simulink model "Fierro_seguidor"  (R2018a)
settings: Solver=ode45  StartTime=0.0  StopTime=1  RelTol=1e-5  EnableMultiTasking=on
undefined symbols (not defined in the file): KIm, Km, KPm, Pm
libraries: simulink x3
settings Model: Creator=dwbertol  LastModifiedBy=bruno
settings DataIOCC: LimitDataPoints=on  SaveFormat=Array  SignalLoggingSaveFormat=ModelDataLogs
settings OptimizationCC: ExpressionDepthLimit=2147483647  LifeSpan=inf
settings DebuggingCC: UnderspecifiedInitializationDetection=Classic  MergeDetectMultiDrivingBlocksExec=none  SolverPrmCheckMsg=warning  FcnCallInpInsideContextMsg=warning  StateNameClashWarn=warning  SFUnexpectedBacktrackingDiag=warning  SFNoUnconditionalDefaultTransitionDiag=warning  SFExecutionAtInitializationDiag=none
settings HardwareCC: ProdBitPerPointer=32  ProdBitPerSizeT=32  ProdBitPerPtrDiffT=32  ProdLargestAtomicFloat=None  ProdIntDivRoundTo=Undefined  ProdEndianess=Unspecified  ProdWordSize=32  ProdHWDeviceType=32-bit Generic
settings ModelReferenceCC: PropagateSignalLabelsOutOfModel=off
settings CodeAppCC: StateflowObjectComments=on
settings GRTTargetCC: TargetLangStandard=C89/C90 (ANSI)  GeneratePreprocessorConditionals=Disable all  CombineOutputUpdateFcns=off  GRTInterface=on
settings ConfigComp: CovMetricSettings=dw  CovHtmlReporting=on  CovSaveCumulativeToWorkspaceVar=on  CovSaveSingleToWorkspaceVar=on  CovExternalEMLEnable=off

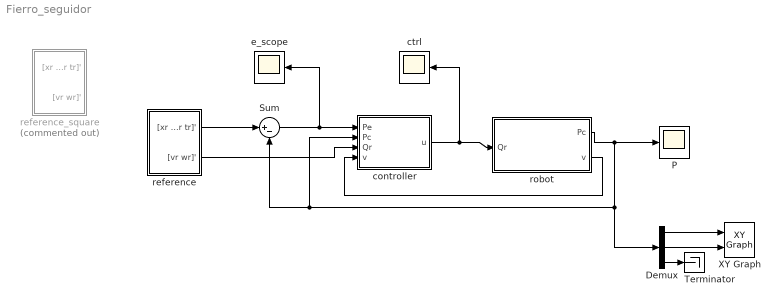
== system Fierro_seguidor ==
  Demux : Demux  Outputs=3
  P : Scope
  Sum : Sum  Inputs=|+-  AccumDataTypeStr=double
  Terminator : Terminator
  XY Graph : simulink/Sinks/XY Graph  xmin=-0.1  xmax=1.1  ymin=-0.1  ymax=1.1  st=Ts
  controller : Subsystem  mask{kx=80, ky=2000, kt=160, k4=100}
  ctrl : Scope
  e_scope : Scope
  reference : Subsystem  mask{vr=1, wr=0, ini=[0 0.2 0], Ts=5e-3}
  reference_square : Subsystem  Commented=on  mask{vr=0.5, wr=0, ini=[0 0 0], Ts=5e-3}
  robot : Subsystem  mask{ini=[0 0 0]'}
  wires:
  controller/1(u) -> robot/1(Qr), ctrl/1
  Demux/3 -> Terminator/1
  Demux/2 -> XY Graph/2
  Demux/1 -> XY Graph/1
  reference/1("[xr yr tr]' ") -> Sum/1
  Sum/1 -> controller/1(Pe), e_scope/1
  reference/2("[vr wr]'") -> controller/3(Qr)
  robot/1(Pc) -> P/1, Demux/1, Sum/2, controller/2(Pc)
  robot/2(v) -> controller/4(v)

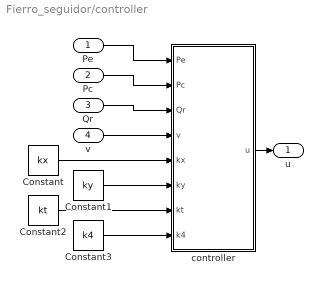
== system Fierro_seguidor/controller ==
  Pe : Inport
  Pc : Inport  Port=2
  Qr : Inport  Port=3
  v : Inport  Port=4
  Constant : Constant  Value=kx
  Constant1 : Constant  Value=ky
  Constant2 : Constant  Value=kt
  Constant3 : Constant  Value=k4
  controller : MATLAB Function  TreatAsAtomicUnit=on
  u : Outport
  wires:
  controller/1(u) -> u/1
  Pe/1 -> controller/1(Pe)
  Pc/1 -> controller/2(Pc)
  Qr/1 -> controller/3(Qr)
  v/1 -> controller/4(v)
  Constant/1 -> controller/5(kx)
  Constant1/1 -> controller/6(ky)
  Constant2/1 -> controller/7(kt)
  Constant3/1 -> controller/8(k4)

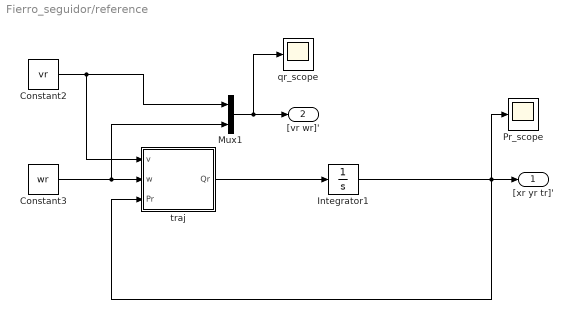
== system Fierro_seguidor/reference ==
  Constant2 : Constant  Value=vr  VectorParams1D=off
  Constant3 : Constant  Value=wr  VectorParams1D=off
  Integrator1 : Integrator  InitialCondition=ini
  Mux1 : Mux  Inputs=2
  Pr_scope : Scope
  qr_scope : Scope
  traj : MATLAB Function  TreatAsAtomicUnit=on
  "[xr yr tr]' " : Outport
  "[vr wr]'" : Outport  Port=2
  wires:
  Integrator1/1 -> Pr_scope/1, traj/3(Pr), "[xr yr tr]' "/1
  Constant3/1 -> Mux1/2, traj/2(w)
  Constant2/1 -> traj/1(v), Mux1/1
  Mux1/1 -> "[vr wr]'"/1, qr_scope/1
  traj/1(Qr) -> Integrator1/1

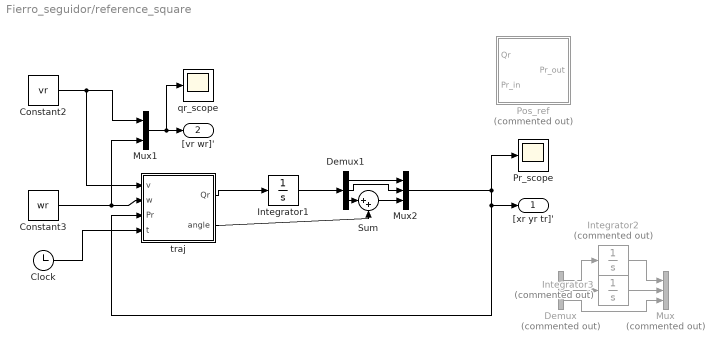
== system Fierro_seguidor/reference_square ==
  Clock : Clock
  Constant2 : Constant  Value=vr  VectorParams1D=off  SampleTime=Ts
  Constant3 : Constant  Value=wr  VectorParams1D=off  SampleTime=Ts
  Demux : Demux  Commented=on  Outputs=3
  Demux1 : Demux  Outputs=3
  Integrator1 : Integrator  InitialCondition=ini
  Integrator2 : Integrator  Commented=on  InitialCondition=ini(1)
  Integrator3 : Integrator  Commented=on  InitialCondition=ini(2)
  Mux : Mux  Commented=on  Inputs=3
  Mux1 : Mux  Inputs=2
  Mux2 : Mux  Inputs=3
  Pos_ref : MATLAB Function  Commented=on  TreatAsAtomicUnit=on
  Pr_scope : Scope
  Sum : Sum  Inputs=|++
  qr_scope : Scope
  traj : MATLAB Function  TreatAsAtomicUnit=on
  "[xr yr tr]' " : Outport
  "[vr wr]'" : Outport  Port=2
  wires:
  Constant2/1 -> traj/1(v), Mux1/1
  Mux1/1 -> "[vr wr]'"/1, qr_scope/1
  traj/1(Qr) -> Integrator1/1
  Constant3/1 -> Mux1/2, traj/2(w)
  Mux2/1 -> "[xr yr tr]' "/1, traj/3(Pr), Pr_scope/1
  Demux/3 -> Mux/3
  Integrator3/1 -> Mux/2
  Demux/1 -> Integrator2/1
  Demux/2 -> Integrator3/1
  Integrator2/1 -> Mux/1
  Integrator1/1 -> Demux1/1
  Demux1/1 -> Mux2/1
  Demux1/2 -> Mux2/2
  Demux1/3 -> Sum/1
  Sum/1 -> Mux2/3
  traj/2(angle) -> Sum/2
  Clock/1 -> traj/4(t)

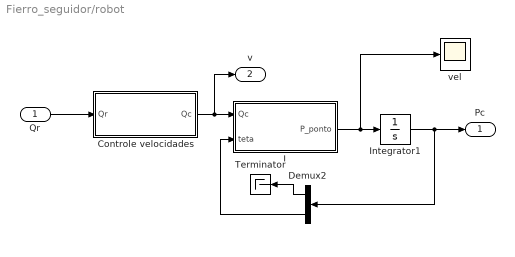
== system Fierro_seguidor/robot ==
  Qr : Inport
  Controle velocidades : Subsystem
  Demux2 : Demux  Outputs=[2 1]
  Integrator1 : Integrator  InitialCondition=ini
  J : MATLAB Function  TreatAsAtomicUnit=on
  Terminator : Terminator
  vel : Scope
  Pc : Outport
  v : Outport  Port=2
  wires:
  J/1(P_ponto) -> vel/1, Integrator1/1
  Integrator1/1 -> Demux2/1, Pc/1
  Demux2/1 -> Terminator/1
  Qr/1 -> Controle velocidades/1(Qr)
  Controle velocidades/1(Qc) -> v/1, J/1(Qc)
  Demux2/2 -> J/2(teta)

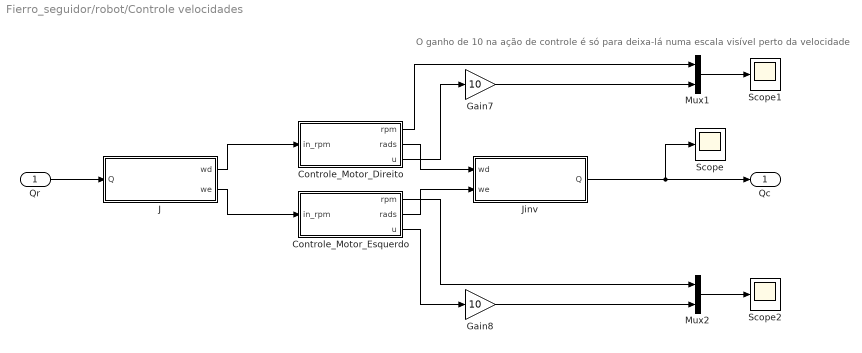
== system Fierro_seguidor/robot/Controle velocidades ==
  note: O ganho de 10 na ação de controle é só para deixa-lá numa escala visível perto da velocidade
  Qr : Inport
  Controle_Motor_Direito : Subsystem
  Controle_Motor_Esquerdo : Subsystem
  Gain7 : Gain  Gain=10
  Gain8 : Gain  Gain=10
  J : MATLAB Function  TreatAsAtomicUnit=on
  Jinv : MATLAB Function  TreatAsAtomicUnit=on
  Mux1 : Mux  Inputs=2
  Mux2 : Mux  Inputs=2
  Scope : Scope
  Scope1 : Scope
  Scope2 : Scope
  Qc : Outport
  wires:
  Gain7/1 -> Mux1/2
  Mux2/1 -> Scope2/1
  Mux1/1 -> Scope1/1
  Gain8/1 -> Mux2/2
  Controle_Motor_Direito/3(u) -> Gain7/1
  Controle_Motor_Direito/1(rpm) -> Mux1/1
  Controle_Motor_Esquerdo/3(u) -> Gain8/1
  Controle_Motor_Esquerdo/1(rpm) -> Mux2/1
  Qr/1 -> J/1(Q)
  J/1(wd) -> Controle_Motor_Direito/1(in_rpm)
  J/2(we) -> Controle_Motor_Esquerdo/1(in_rpm)
  Controle_Motor_Direito/2(rads) -> Jinv/1(wd)
  Controle_Motor_Esquerdo/2(rads) -> Jinv/2(we)
  Jinv/1(Q) -> Scope/1, Qc/1

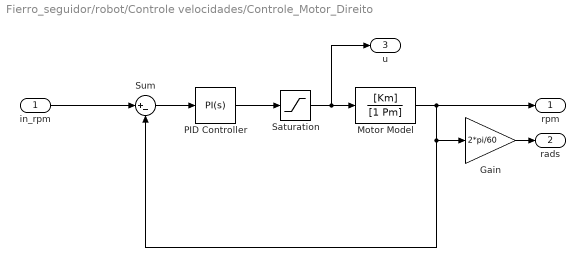
== system Fierro_seguidor/robot/Controle velocidades/Controle_Motor_Direito ==
  in_rpm : Inport
  Gain : Gain  Gain=2*pi/60
  Motor Model : TransferFcn  Numerator=[Km]  Denominator=[1 Pm]
  PID Controller : simulink/Continuous/PID Controller  Controller=PI  TimeDomain=Continuous-time  SampleTime=-1  IntegratorMethod=Forward Euler  FilterMethod=Forward Euler  Form=Parallel  UseFilter=on  ControllerParametersSource=internal  P=KPm  I=KIm  D=0  N=0  InitialConditionSource=internal  InitialConditionForIntegrator=0  InitialConditionForFilter=0  ExternalReset=none  LimitOutput=off  UpperSaturationLimit=inf  LowerSaturationLimit=-inf  LinearizeAsGain=on  AntiWindupMode=none  Kb=1  TrackingMode=off  Kt=1  PParamMin=[]  PParamMax=[]  IParamMin=[]  IParamMax=[]  DParamMin=[]  DParamMax=[]  NParamMin=[]  NParamMax=[]  KbParamMin=[]  KbParamMax=[]  KtParamMin=[]  KtParamMax=[]  POutMin=[]  POutMax=[]  IOutMin=[]  IOutMax=[]  DOutMin=[]  DOutMax=[]  NOutMin=[]  NOutMax=[]  KbOutMin=[]  KbOutMax=[]  KtOutMin=[]  KtOutMax=[]  IntegratorOutMin=[]  IntegratorOutMax=[]  FilterOutMin=[]  FilterOutMax=[]  SumOutMin=[]  SumOutMax=[]  SumI1OutMin=[]  SumI1OutMax=[]  SumI2OutMin=[]  SumI2OutMax=[]  SumI3OutMin=[]  SumI3OutMax=[]  SumDOutMin=[]  SumDOutMax=[]  SaturationOutMin=[]  SaturationOutMax=[]  IntegratorContinuousStateAttributes=''  IntegratorStateMustResolveToSignalObject=off  IntegratorRTWStateStorageClass=Auto  FilterContinuousStateAttributes=''  FilterStateMustResolveToSignalObject=off  FilterRTWStateStorageClass=Auto  DifferentiatorICPrevScaledInput=0  DifferentiatorOutMin=[]  DifferentiatorOutMax=[]  FilterDiffOutCoefMin=[]  FilterDiffOutCoefMax=[]  SumDenOutMin=[]  SumDenOutMax=[]  SumNumOutMin=[]  SumNumOutMax=[]  ReciprocalOutMin=[]  ReciprocalOutMax=[]  DivideOutMin=[]  DivideOutMax=[]  TunerSelectOption=Transfer Function Based (PID Tuner App)
  Saturation : Saturate  UpperLimit=100  LowerLimit=-100
  Sum : Sum  Inputs=|+-
  rpm : Outport
  rads : Outport  Port=2
  u : Outport  Port=3
  wires:
  PID Controller/1 -> Saturation/1
  Motor Model/1 -> rpm/1, Gain/1, Sum/2
  Saturation/1 -> u/1, Motor Model/1
  Sum/1 -> PID Controller/1
  in_rpm/1 -> Sum/1
  Gain/1 -> rads/1

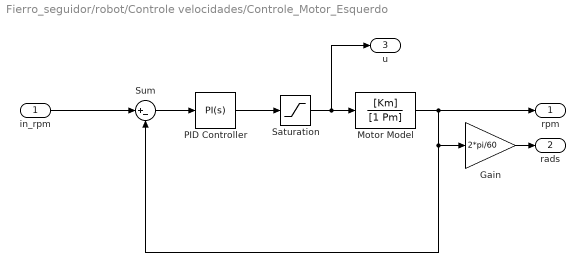
== system Fierro_seguidor/robot/Controle velocidades/Controle_Motor_Esquerdo ==
  in_rpm : Inport
  Gain : Gain  Gain=2*pi/60
  Motor Model : TransferFcn  Numerator=[Km]  Denominator=[1 Pm]
  PID Controller : simulink/Continuous/PID Controller  Controller=PI  TimeDomain=Continuous-time  SampleTime=-1  IntegratorMethod=Forward Euler  FilterMethod=Forward Euler  Form=Parallel  UseFilter=on  ControllerParametersSource=internal  P=KPm  I=KIm  D=0  N=0  InitialConditionSource=internal  InitialConditionForIntegrator=0  InitialConditionForFilter=0  ExternalReset=none  LimitOutput=off  UpperSaturationLimit=inf  LowerSaturationLimit=-inf  LinearizeAsGain=on  AntiWindupMode=none  Kb=1  TrackingMode=off  Kt=1  PParamMin=[]  PParamMax=[]  IParamMin=[]  IParamMax=[]  DParamMin=[]  DParamMax=[]  NParamMin=[]  NParamMax=[]  KbParamMin=[]  KbParamMax=[]  KtParamMin=[]  KtParamMax=[]  POutMin=[]  POutMax=[]  IOutMin=[]  IOutMax=[]  DOutMin=[]  DOutMax=[]  NOutMin=[]  NOutMax=[]  KbOutMin=[]  KbOutMax=[]  KtOutMin=[]  KtOutMax=[]  IntegratorOutMin=[]  IntegratorOutMax=[]  FilterOutMin=[]  FilterOutMax=[]  SumOutMin=[]  SumOutMax=[]  SumI1OutMin=[]  SumI1OutMax=[]  SumI2OutMin=[]  SumI2OutMax=[]  SumI3OutMin=[]  SumI3OutMax=[]  SumDOutMin=[]  SumDOutMax=[]  SaturationOutMin=[]  SaturationOutMax=[]  IntegratorContinuousStateAttributes=''  IntegratorStateMustResolveToSignalObject=off  IntegratorRTWStateStorageClass=Auto  FilterContinuousStateAttributes=''  FilterStateMustResolveToSignalObject=off  FilterRTWStateStorageClass=Auto  DifferentiatorICPrevScaledInput=0  DifferentiatorOutMin=[]  DifferentiatorOutMax=[]  FilterDiffOutCoefMin=[]  FilterDiffOutCoefMax=[]  SumDenOutMin=[]  SumDenOutMax=[]  SumNumOutMin=[]  SumNumOutMax=[]  ReciprocalOutMin=[]  ReciprocalOutMax=[]  DivideOutMin=[]  DivideOutMax=[]  TunerSelectOption=Transfer Function Based (PID Tuner App)
  Saturation : Saturate  UpperLimit=100  LowerLimit=-100
  Sum : Sum  Inputs=|+-
  rpm : Outport
  rads : Outport  Port=2
  u : Outport  Port=3
  wires:
  PID Controller/1 -> Saturation/1
  Saturation/1 -> u/1, Motor Model/1
  Sum/1 -> PID Controller/1
  in_rpm/1 -> Sum/1
  Motor Model/1 -> rpm/1, Gain/1, Sum/2
  Gain/1 -> rads/1

== matlab function Fierro_seguidor/reference_square/traj ==
  data: v input size=1; w input; Pr input size=3; Qr output size=3; angle output size=1; t input
function [Qr, angle] = fcn(v, w, Pr, t)
 
 if (Pr(1) <= 1) && (Pr(2) <= 0)
     Pr(3) = 0;
 else if (Pr(1) >= 1) && (Pr(2) <= 1)
        Pr(3) = pi/2;
     else if (Pr(1) >= 1) && (Pr(2) >= 1)
             Pr(3) = pi;
         else if (Pr(1) <= 0) && (Pr(2) >= 1)
                 Pr(3) = 270*pi/180;
             end 
         end
     end
 end
 
 Qr = [cos(Pr(3)) 0; sin(Pr(3)) 0; 0 1]*[v; w];
 angle = Pr(3);
 
end

== matlab function Fierro_seguidor/robot/Controle velocidades/J ==
  data: Q input; wd output; we output
function [wd, we] = fcn(Q)
% Dados do robô
r = 16e-3;      % Raio da roda
a = 69e-3;      % Distância do centro do robô até o centro das rodas

w_mot_rpm = (60/(2*pi))*[1/r a/r; 1/r -a/r]*Q;   % o 60/(2pi) é pra converter p/ rpm
wd = w_mot_rpm(1);
we = w_mot_rpm(2);

== matlab function Fierro_seguidor/robot/Controle velocidades/Jinv ==
  data: wd input; Q output; we input
function Q = fcn(wd, we)
% Dados do robô
r = 16e-3;      % Raio da roda
a = 69e-3;      % Distância do centro do robô até o centro das rodas

Q = (r/2)*[1 1; 1/a -1/a]*[wd; we];

== matlab function Fierro_seguidor/controller/controller ==
  data: Pe input size=3; Pc input size=3; Qr input size=2; v input size=2; u output size=2; kx input; ky input; kt input; k4 input
function u = fcn(Pe,Pc,Qr,v,kx,ky,kt,k4)

e = [cos(Pc(3)) sin(Pc(3)) 0; -sin(Pc(3)) cos(Pc(3)) 0; 0 0 1]*Pe;
%  Pe(1) = 0;  %essa linha é um caso a parte (para o seguidor de linha)

Qc = [Qr(1)*cos(e(3))+kx*e(1);Qr(2)+ky*Qr(1)*e(2)+kt*Qr(1)*sin(e(3))];
 
ep = [v(2)*e(2)-v(1)+Qr(1)*cos(e(3));-v(2)*e(1)+Qr(1)*sin(e(3));Qr(2)-v(2)];
Qcp = [kx 0 -Qr(1)*sin(e(3)); 0 ky*Qr(1) kt*Qr(1)*cos(e(3))]*ep;
 
u = k4*(Qc-v) + Qcp;

 
end

== matlab function Fierro_seguidor/robot/J ==
  data: Qc input size=2; P_ponto output size=3; teta input size=1
function P_ponto = fcn(Qc, teta)

P_ponto = [Qc(1)*cos(teta); Qc(1)*sin(teta); Qc(2)]; %[Vx, Vy, Vteta];

== matlab function Fierro_seguidor/reference_square/Pos_ref ==
  data: Qr input; Pr_out output; Pr_in input
function Pr_out = fcn(Qr, Pr_in)
    Pr_out = Qr;
    Pr_out(1) = Pr_in(1) + Qr(1)*Ts;
    Pr_out(2) = Pr_in(2) + Qr(2)*Ts;
    Pr_out(3) = Qr(3);
 
end

== matlab function Fierro_seguidor/reference/traj ==
  data: v input; w input; Pr input; Qr output
function Qr = fcn(v, w, Pr)

 Qr = [cos(Pr(3)) 0; sin(Pr(3)) 0; 0 1]*[v; w];
 
end
